simulink model "HW5_Simulink"  (R2019b)
settings: Solver=FixedStepAuto  StartTime=0.0  StopTime=10  RelTol=1e-3
InitFcn:
  | load('BusDefinitions.mat')
values from neighbouring files (symbols this model uses):
  q = states(:,5)    [HW5.m]
  r = states(:,6)    [HW5.m]
undefined symbols (not defined in the file or in its folder): A_eval, B_eval, C_eval, codertarget, D_eval, Discrete, Time, Ts
libraries: ctrlSharedLib x1
settings Model: ExtModeTrigDuration=80  Creator=Sankalp Bhan  LastModifiedBy=cwhipp
settings OptimizationCC: PassReuseOutputArgsThreshold=0  MaxStackSize=64
settings DebuggingCC: ParameterTunabilityLossMsg=error  ArithmeticOperatorsInVariantConditions=warning
settings HardwareCC: ProdBitPerPointer=32  ProdBitPerSizeT=32  ProdBitPerPtrDiffT=32  ProdLargestAtomicInteger=Long  ProdWordSize=32  ProdHWDeviceType=ARM Compatible->ARM 9  UseEmbeddedCoderFeatures=off
settings SFSimCC: SimUseLocalCustomCode=off  MATLABDynamicMemAlloc=off
settings RTWCC: SystemTargetFile=ert.tlc  HardwareBoard=PARROT Mambo  TLCOptions="-aInlineSetEventsForThisBaseRateFcn=TLC_FALSE -aSuppressMultiTaskScheduler=TLC_FALSE   -aRateBasedStepFcn=1"  TemplateMakefile=ert_default_tmf  GenerateReport=on  RTWUseLocalCustomCode=off  Toolchain=Sourcery G++ Lite GNU Toolchain for Drones  LaunchReport=on
settings CodeAppCC: ForceParamTrailComments=on  OperatorAnnotations=on  StateflowObjectComments=on
settings ERTTargetCC: ERTCustomFileBanners=off  MatFileLogging=on  SupportContinuousTime=on  SupportNonInlinedSFcns=on  RemoveResetFunc=off  ModelStepFunctionPrototypeControlCompliant=off

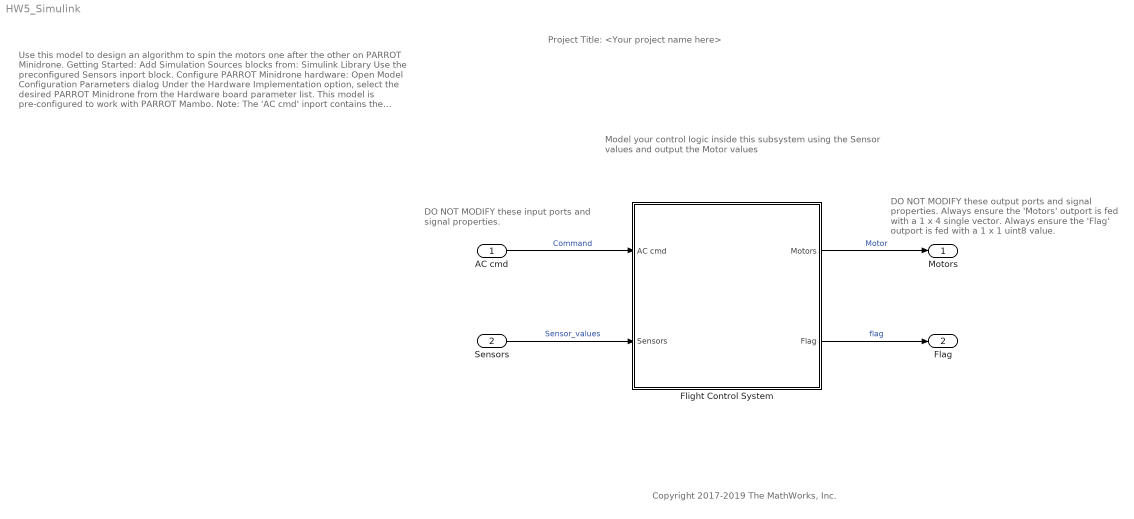
== system HW5_Simulink ==
  note: Model your control logic inside this subsystem
      | using the Sensor values and output the
      | Motor values
  note: DO NOT MODIFY these output ports
      | and signal properties.
      |
      |
      |
      | Always ensure the 'Motors' outport
      | is fed with a 1 x 4 single vector.
      |
      |
      |
      |
      |
      | Always ensure the 'Flag' outport is
      | fed with a 1 x 1 uint8 value.
  note: DO NOT MODIFY these input
      | ports and signal properties.
  note: Copyright 2017-2019 The MathWorks, Inc.
  note: Use this model to design an algorithm to spin the motors one
      | after the other on PARROT Minidrone.
      |
      | Getting Started:
      |
      | Add Simulation Sources blocks from:
      | Simulink Library
      | Use the preconfigured Sensors inport block.
      |
      | Configure PARROT Minidrone hardware:
      |
      | Open Model Configuration Parameters dialog
      |
      | Under the Hardware Implementation option, select the desired
      | PARROT Minidrone from the Hardware board parameter list.
      |
      | This model is pre-configured to work with PARROT Mambo.
      |
      | Note:
      |
      | The 'AC cmd' inport contains the position and orientation
      | reference signals information.
      | The 'Sensors' inport contains data from accelerometer,
      | gyroscope, ultrasonic, pressure and optical flow data.
      | The 'Flag' outport can be used to model an error condition
      | which stops the drone.
      | The 'Motors' outport is fed with the speed values of the 4 motors.
      | Learn more:
      |
      | Simulink Subsystem
      | Simulink Buses
  note: Project Title: <Your project name here>
  AC cmd : Inport  OutDataTypeStr=Bus: CommandBus  BusOutputAsStruct=on
  Sensors : Inport  Port=2  OutDataTypeStr=Bus: SensorsBus  BusOutputAsStruct=on
  Flight Control System : Subsystem  InitFcn=codertarget.parrot.internal.fcsSubsystemCallback(gcb);
  Motors : Outport  OutDataTypeStr=single  PortDimensions=[1 4]  VectorParamsAs1DForOutWhenUnconnected=off
  Flag : Outport  Port=2  OutDataTypeStr=uint8  PortDimensions=1  VectorParamsAs1DForOutWhenUnconnected=off
  wires:
  Flight Control System/1(Motors) -> Motors/1  "Motor"
  AC cmd/1 -> Flight Control System/1(AC cmd)  "Command"
  Sensors/1 -> Flight Control System/2(Sensors)  "Sensor_values"
  Flight Control System/2(Flag) -> Flag/1  "flag"

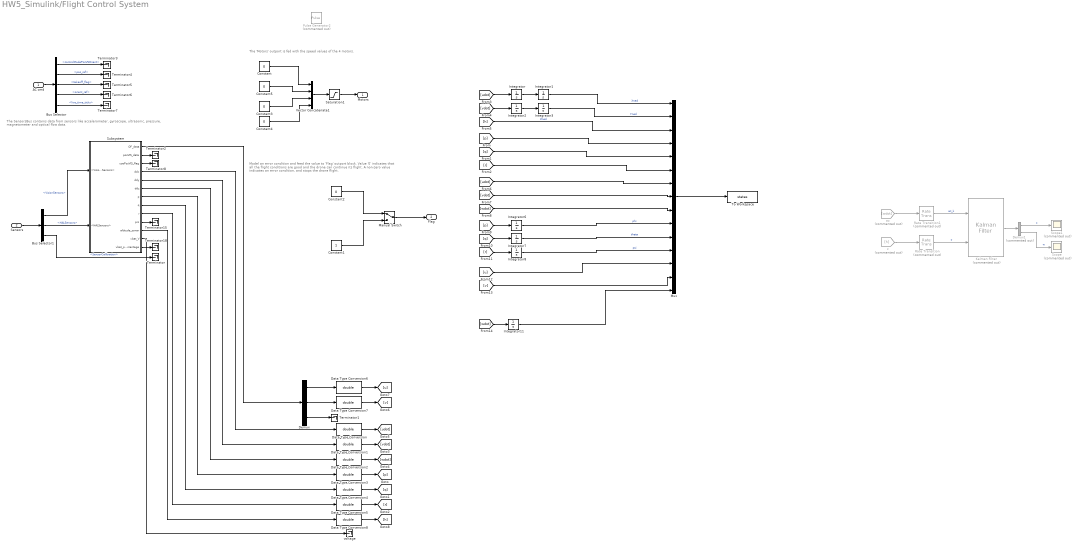
== system HW5_Simulink/Flight Control System ==
  note: The 'Motors' outport is fed with the speed values of the 4 motors.
  note: Model an error condition and feed the value to 'Flag' outport block.
      | Value '0' indicates that all the flight conditions are good and the drone
      | can continue its flight.
      | A non-zero value indicates an error condition, and stops the drone
      | flight.
  note: The SensorsBus contains data from sensors like
      | accelerometer, gyroscope, ultrasonic, pressure,
      | magnetometer and optical flow data.
  AC cmd : Inport
  Sensors : Inport  Port=2
  Bus Selector : BusSelector  OutputSignals=controlModePosVSOrient,pos_ref,takeoff_flag,orient_ref,live_time_ticks
  Bus Selector1 : BusSelector  OutputSignals=VisionSensors,HALSensors,SensorCalibration
  Constant{,3..5} (4 alike) : Constant  Value=0  SampleTime=0.005
  Constant1 : Constant  OutDataTypeStr=uint8
  Constant2 : Constant  Value=0  OutDataTypeStr=uint8
  Data Type Conversion{,1..8} (9 alike) : DataTypeConversion  OutDataTypeStr=double
  Demux : Demux  Outputs=3
  Demux1 : Demux  Commented=on  Outputs=2
  Integrator{,1..3,6..8,11} (8 alike) : Integrator
  Kalman Filter : ctrlSharedLib/Kalman Filter  Commented=on  TimeDomain=Discrete-Time  UseCurrentEstimator=on  ModelSource=Individual A, B, C, D matrices  ModelSourceVariable=ss(0.95,1,1,0,1)  A=A_eval  B=B_eval  C=C_eval  D=D_eval  NumberOfStates=1  NumberOfInputs=1  NumberOfOutputs=1  InitialEstimateSource=Dialog  X0=[0;0 ]  P0=10  UseK=off  UseGH=off  NumberOfProcessNoiseInputs=1  G=1  TimeInvariantG=on  H=0  TimeInvariantH=on  Q=[0 0 ; 0 1]*q;  TimeInvariantQ=on  R=r;  TimeInvariantR=on  N=0  TimeInvariantN=on  AddInputPort=on  AddEnablePort=off  OutputEstimatedY=off  OutputP=off  Ts=-1
      settings: SourceProductBaseCode=CT
  Manual Switch : ManualSwitch
  Mux : Mux  Inputs=15
  Pulse Generator2 : DiscretePulseGenerator  Commented=on  Amplitude=400  Period=1600  PulseWidth=400  PhaseDelay=1200  SampleTime=Ts
  Rate Transition : RateTransition  Commented=on  OutPortSampleTime=0.005
  Rate Transition1 : RateTransition  Commented=on  OutPortSampleTime=0.005
  Saturation1 : Saturate  UpperLimit=500  LowerLimit=0  OutDataTypeStr=single
  Scope : Scope  Commented=on
  Scope1 : Scope  Commented=on
  Subsystem : Subsystem
  Terminator{,1..8,15,18} (11 alike) : Terminator
  To Workspace : ToWorkspace  VariableName=states  SaveFormat=Structure With Time  SampleTime=-1
  Vector Concatenate1 : Concatenate  NumInputs=4
  az : From  Commented=on  GotoTag=wdot
  voltage : Terminator
  z : From  Commented=on  GotoTag=h
  Motors : Outport  VectorParamsAs1DForOutWhenUnconnected=off
  Flag : Outport  Port=2  VectorParamsAs1DForOutWhenUnconnected=off
  wires:
  AC cmd/1 -> Bus Selector/1
  Sensors/1 -> Bus Selector1/1
  Bus Selector/1 -> Terminator3/1  "<controlModePosVSOrient>"
  Bus Selector/2 -> Terminator4/1  "<pos_ref>"
  Bus Selector/3 -> Terminator5/1  "<takeoff_flag>"
  Bus Selector/4 -> Terminator6/1  "<orient_ref>"
  Bus Selector/5 -> Terminator7/1  "<live_time_ticks>"
  Manual Switch/1 -> Flag/1
  Constant2/1 -> Manual Switch/1
  Constant1/1 -> Manual Switch/2
  Vector Concatenate1/1 -> Saturation1/1
  Constant/1 -> Vector Concatenate1/1
  Constant4/1 -> Vector Concatenate1/4
  Constant5/1 -> Vector Concatenate1/2
  Constant3/1 -> Vector Concatenate1/3
  Saturation1/1 -> Motors/1
  Bus Selector1/1 -> Subsystem/1(<VisionSensors>)  "<VisionSensors>"
  Bus Selector1/2 -> Subsystem/2(<HALSensors>)  "<HALSensors>"
  Bus Selector1/3 -> Terminator/1  "<SensorCalibration>"
  Subsystem/1(OF_data) -> Demux/1
  Subsystem/2(posVIS_data) -> Terminator2/1
  Subsystem/3(usePosVIS_flag) -> Terminator8/1
  Subsystem/10(prs) -> Terminator15/1
  Subsystem/11(altitude_sonar) -> Data Type Conversion8/1
  Subsystem/13(vbat_percentage) -> Terminator18/1
  [udot] -> Integrator/1
  Integrator/1 -> Integrator1/1
  Integrator2/1 -> Integrator3/1
  [vdot] -> Integrator2/1
  [r] -> Integrator8/1
  [p] -> Integrator6/1
  [q] -> Integrator7/1
  [wdot] -> Integrator11/1
  [h] -> Mux/3  "Zned"
  Integrator3/1 -> Mux/2  "Yned"
  Integrator1/1 -> Mux/1  "Xned"
  [p] -> Mux/4
  [q] -> Mux/5
  Subsystem/4(ddx) -> Data Type Conversion/1
  Data Type Conversion/1 -> [udot]
  Subsystem/5(ddy) -> Data Type Conversion1/1
  Data Type Conversion1/1 -> [vdot]
  Subsystem/6(ddz) -> Data Type Conversion2/1
  Data Type Conversion2/1 -> [wdot]
  Subsystem/7(p) -> Data Type Conversion3/1
  Data Type Conversion3/1 -> [p]
  Subsystem/8(q) -> Data Type Conversion4/1
  Data Type Conversion4/1 -> [q]
  Subsystem/9(r) -> Data Type Conversion5/1
  Data Type Conversion5/1 -> [r]
  Data Type Conversion7/1 -> [v]
  Data Type Conversion6/1 -> [u]
  Demux/1 -> Data Type Conversion6/1
  Demux/2 -> Data Type Conversion7/1
  Demux/3 -> Terminator1/1
  Data Type Conversion8/1 -> [h]
  Subsystem/12(vbat_V) -> voltage/1
  Mux/1 -> To Workspace/1
  Integrator6/1 -> Mux/10  "phi"
  Integrator7/1 -> Mux/11  "theta"
  Integrator8/1 -> Mux/12  "psi"
  Integrator11/1 -> Mux/15
  [udot] -> Mux/7
  [vdot] -> Mux/8
  [wdot] -> Mux/9
  [r] -> Mux/6
  [u] -> Mux/13
  [v] -> Mux/14
  Demux1/2 -> Scope/1  "w"
  Rate Transition1/1 -> Kalman Filter/1  "az_k"
  Rate Transition/1 -> Kalman Filter/2  "y"
  Kalman Filter/1 -> Demux1/1
  Demux1/1 -> Scope1/1  "z"
  az/1 -> Rate Transition1/1
  z/1 -> Rate Transition/1

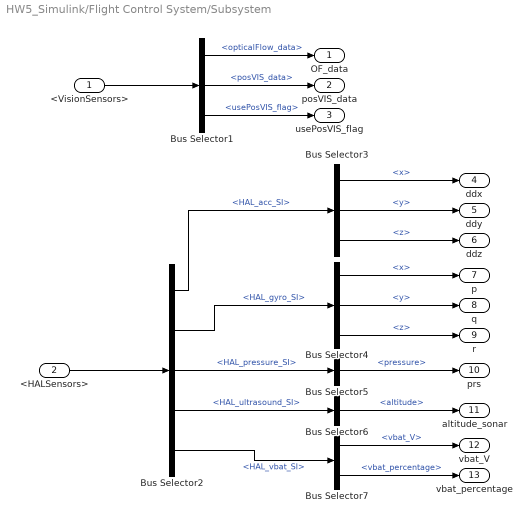
== system HW5_Simulink/Flight Control System/Subsystem ==
  <VisionSensors> : Inport
  <HALSensors> : Inport  Port=2
  Bus Selector1 : BusSelector  OutputSignals=opticalFlow_data,posVIS_data,usePosVIS_flag
  Bus Selector2 : BusSelector  OutputSignals=HAL_acc_SI,HAL_gyro_SI,HAL_pressure_SI,HAL_ultrasound_SI,HAL_vbat_SI
  Bus Selector3 : BusSelector  OutputSignals=x,y,z
  Bus Selector4 : BusSelector  OutputSignals=x,y,z
  Bus Selector5 : BusSelector  OutputSignals=pressure
  Bus Selector6 : BusSelector  OutputSignals=altitude
  Bus Selector7 : BusSelector  OutputSignals=vbat_V,vbat_percentage
  OF_data : Outport  VectorParamsAs1DForOutWhenUnconnected=off
  posVIS_data : Outport  Port=2  VectorParamsAs1DForOutWhenUnconnected=off
  usePosVIS_flag : Outport  Port=3  VectorParamsAs1DForOutWhenUnconnected=off
  ddx : Outport  Port=4  VectorParamsAs1DForOutWhenUnconnected=off
  ddy : Outport  Port=5  VectorParamsAs1DForOutWhenUnconnected=off
  ddz : Outport  Port=6  VectorParamsAs1DForOutWhenUnconnected=off
  p : Outport  Port=7  VectorParamsAs1DForOutWhenUnconnected=off
  q : Outport  Port=8  VectorParamsAs1DForOutWhenUnconnected=off
  r : Outport  Port=9  VectorParamsAs1DForOutWhenUnconnected=off
  prs : Outport  Port=10  VectorParamsAs1DForOutWhenUnconnected=off
  altitude_sonar : Outport  Port=11  VectorParamsAs1DForOutWhenUnconnected=off
  vbat_V : Outport  Port=12  VectorParamsAs1DForOutWhenUnconnected=off
  vbat_percentage : Outport  Port=13  VectorParamsAs1DForOutWhenUnconnected=off
  wires:
  <VisionSensors>/1 -> Bus Selector1/1
  <HALSensors>/1 -> Bus Selector2/1
  Bus Selector1/1 -> OF_data/1  "<opticalFlow_data>"
  Bus Selector1/2 -> posVIS_data/1  "<posVIS_data>"
  Bus Selector1/3 -> usePosVIS_flag/1  "<usePosVIS_flag>"
  Bus Selector2/1 -> Bus Selector3/1  "<HAL_acc_SI>"
  Bus Selector2/2 -> Bus Selector4/1  "<HAL_gyro_SI>"
  Bus Selector2/3 -> Bus Selector5/1  "<HAL_pressure_SI>"
  Bus Selector2/4 -> Bus Selector6/1  "<HAL_ultrasound_SI>"
  Bus Selector2/5 -> Bus Selector7/1  "<HAL_vbat_SI>"
  Bus Selector3/1 -> ddx/1  "<x>"
  Bus Selector3/2 -> ddy/1  "<y>"
  Bus Selector3/3 -> ddz/1  "<z>"
  Bus Selector4/2 -> q/1  "<y>"
  Bus Selector4/1 -> p/1  "<x>"
  Bus Selector4/3 -> r/1  "<z>"
  Bus Selector5/1 -> prs/1  "<pressure>"
  Bus Selector6/1 -> altitude_sonar/1  "<altitude>"
  Bus Selector7/1 -> vbat_V/1  "<vbat_V>"
  Bus Selector7/2 -> vbat_percentage/1  "<vbat_percentage>"
